simulink model "LQR"  (R2015a)
settings: Solver=ode45  StartTime=0.0  StopTime=10.0  FixedStep=0.02  RelTol=1e-3
values from neighbouring files (symbols this model uses):
  A = [0,1,0;(mb*lb+mw*l)*g/(Ib+mw*(l^2)),-Cb/(Ib+mw*(l^2)),Cw/(Ib+mw*(l^2));-(mb*lb+mw*l)*g/(Ib+mw*(l^2)),Cb/(Ib+mw*(l^2)),-Cw*(Ib+Iw+mw*(l^2))/(Ib+mw*(l^2))/Iw]    [CubliFunction.m]
  B = [0;-Km/(Ib+mw*(l^2));Km*(Ib+Iw+mw*(l^2))/(Ib+mw*(l^2))/Iw]    [CubliFunction.m]
  K1 = K(1,1)    [CubliFunction.m]
  K2 = K(1,2)    [CubliFunction.m]
  K3 = K(1,3)    [CubliFunction.m]
settings Model: Creator=Remy  LastModifiedBy=Remy

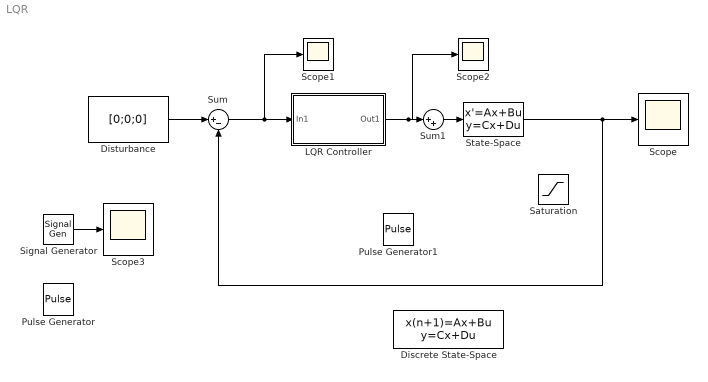
== system LQR ==
  Discrete State-Space : DiscreteStateSpace  SampleTime=0.05
  Disturbance : Constant  Value=[0;0;0]
  LQR Controller : Subsystem  mask(LQR Controller){K1=K1, K2=K2, K3=K3}
  Pulse Generator : DiscretePulseGenerator  PulseType=Time based  Period=10  PulseWidth=5
  Pulse Generator1 : DiscretePulseGenerator  PulseType=Time based  Period=10  PulseWidth=5
  Saturation : Saturate
  Scope{,1..3} (4 alike) : Scope
      Scope settings: ShowLegends=on  SampleTime=0.02
      Scope2 settings: TimeRange=7.524253332715403e-05  YMin=-182.7912760416666  YMax=-182.7734635416666  SaveName=ScopeData2
      Scope3 settings: ShowLegends=on  SaveName=ScopeData3  SampleTime=0.02
  Signal Generator : SignalGenerator  WaveForm=square  Units=rad/sec
  State-Space : StateSpace  A=A  B=B  C=eye(3)  D=zeros(3,1)  X0=[0.1;0;0]  ContinuousStateAttributes={'a', 'b', 'c'}
  Sum : Sum  Inputs=|+-
  Sum1 : Sum  Inputs=|++
  wires:
  Disturbance/1 -> Sum/1
  LQR Controller/1(Out1) -> Sum1/1, Scope2/1
  Sum/1 -> Scope1/1, LQR Controller/1(In1)
  State-Space/1 -> Sum/2, Scope/1
  Signal Generator/1 -> Scope3/1
  Sum1/1 -> State-Space/1

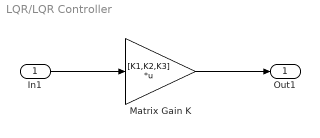
== system LQR/LQR Controller ==
  In1 : Inport
  Matrix Gain K : Gain  Gain=[K1,K2,K3]  Multiplication=Matrix(K*u)
  Out1 : Outport
  wires:
  In1/1 -> Matrix Gain K/1
  Matrix Gain K/1 -> Out1/1
